simulink library "SMC"  (R2021b)
settings: Solver=VariableStepAuto  StartTime=0.0  StopTime=10.0  RelTol=1e-3
values from neighbouring files (symbols this model uses):
  Ao = At    [SMCDesign_init.m]    (also in SMCDesign_initIA.m)
  Bo = Bv    [SMCDesign_init.m]    (also in SMCDesign_initIA.m)
  CA = pinv(B2)    [SMCCanForm.m]
  Co = Ct    [SMCDesign_init.m]    (also in SMCDesign_initIA.m)
  F = -eye(2)    [Example_init.m]
  Lam_inv = inv(Lam)    [SMCDesign_init.m]    (also in SMCDesign_initIA.m)
  P = lyap(Phi',eye(mm))    [contliaCA2.m]
  To_inv = inv(Tr)    [SMCDesign_init.m]    (also in SMCDesign_initIA.m)
undefined symbols (not defined in the file or in its folder): G, Gl, Gn, P2
libraries: $bdroot x2
settings Model: Creator=lev201  LastModifiedBy=w.schwamm
settings SolverCC: AlgebraicLoopSolver=TrustRegion
settings DataIOCC: ReturnWorkspaceOutputs=off
settings DebuggingCC: SFMachineParentedDataDiag=warning  ArithmeticOperatorsInVariantConditions=warning
settings SFSimCC: SimUseLocalCustomCode=off  CustomCodeUndefinedFunction=UseInterfaceOnly
settings RTWCC: RTWUseLocalCustomCode=off

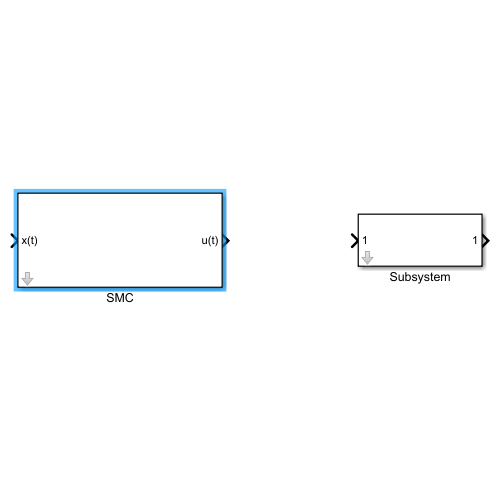
[thumbnail: Simulink's stored preview of the top-level diagram]
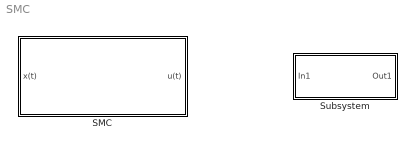
== system SMC ==
  SMC : Subsystem  mask(Sliding Mode Controller){ia=off, obs=off, adpt=off, shs=off, shxo=off, shadpt=off, A=eye(2), B=eye(2), Cc=eye(2), x0=zeros(1,2), obstype=Walcott_Zak, z0=zeros(1,2), Q=eye(2), rho=1, delta=0.01, eps=0, C0=1, PC=1, K0=1, PK=1, Qi=eye(2), Fil=on, Filter=eye(2), FRt=on, rhoo=1, deltao=0.01, epso=0}
      mask prompts: ia "Integral Action"; obs "Observer"; adpt "Adaptive"; shs "Show s(t)"; shxo "Show xo(t)"; shadpt "Show ap(t)"; A "System Matrix (A):"; B "Input Matrix (B):"; Cc "Output Matrix (C):"; x0 "Initial State Vector (x0):"; obstype "Observer Type:"; z0 "Initial State Vector (z0):"; Q "State Weighting Matrix (Q):"; rho "Sliding mode gain (rho):"; delta "Sigmoidal Approximation (delta):"; eps "Boundary Layer Thickness (eps):"; C0 "Initial guess of C:"; PC "Learning rate of C estimator:"; K0 "Initial guess of K:"; PK "Learning rate of K estimator:"; Qi "Integral Action Weighting Matrix (Qi):"; Fil "Pre-Filter Reference Signal"; FRt "Show Filtered R(t)"; rhoo "Sliding mode gain (rhoo):"; deltao "Sigmoidal Approximation (deltao):"; epso "Boundary Layer Thickness (epso):"
      mask help:
      | Sliding Mode Controller with optional observer design
      | Quadratic Minimisation based Sliding Mode Controller with Integral Action
      | If system is over-actuated Control Allocation is automatically used
      mask init:
      | % disp(['shs:' get_param(gcb,'shs')])
      | % clc
      | int=get_param(gcb, 'ia');
      | Shs=get_param(gcb, 'shs');
      | Shxo=get_param(gcb, 'shxo');
      | Fil=get_param(gcb, 'fil');
      | FRT=get_param(gcb, 'FRt');
      | SAD=get_param(gcb, 'shadpt');
      | AD=get_param(gcb, 'adpt');
      | Obs=get_param(gcb, 'obs');
      | 
      | if ~bdIsLibrary(bdroot)
      |     disp('outside lib')
      | else
      |     disp('inside lib')
      | end
      | 
      | [nn mm]=size(B);
      | 
      | % observer is used, if the output matrix does not have full rank
      | % or the flag is set explicitly
      | 
      | % get current number of outports
      | f = Simulink.FindOptions('SearchDepth',1);
      | % num_in=length(Simulink.findBlocksOfType(gcb, 'Inport',f));
      | % num_out=length(Simulink.findBlocksOfType(gcb, 'Outport',f));
      | %fprintf('%d',length(Simulink.findBlocksOfType(gcb, 'Inport',f)))
      | 
      | if strcmp(AD, 'on')
      |     rho=0;
      |     ADPT=1;
      | else
      |     ADPT=0;
      | end
      | 
      | if strcmp(AD, 'on') && strcmp(SAD, 'on')
      |     if strcmp(get_param([gcb '/ap(t)'], 'BlockType'), 'Terminator')
      |         replace([gcb '/ap(t)'], 'built-in/Outport');
      |         num_out=length(Simulink.findBlocksOfType(gcb, 'Outport',f));
      |         set_param([gcb '/ap(t)'],'Port',num2str(num_out));
      |     end
      | else
      |     if strcmp(get_param([gcb '/ap(t)'], 'BlockType'),'Outport')
      |         replace([gcb '/ap(t)'], 'built-in/Terminator')
      |     end
      | end
      | 
      | switch int
      |     case 'off'
      |         [L, P, Lam_inv, S, E, CA,...
      |             Ao, Bo, Co, To_inv, G, F, Gl, Gn, P2]=SMCDesign_init(A, B, Cc, Q);
      |         INTs=0;
      |         ll=size(S,1);
      |         %C=zeros(ll, nn);
      |         L=[zeros(ll, ll) L];
      |         S=[zeros(ll, ll) S];
      |         Sr=zeros(ll, ll);
      |         Lr=[zeros(ll, ll)];
      |         Lrdot=[zeros(ll, ll)];
      |     case 'on'
      |         nn=size(Q,1);
      |         ll=size(Qi,1);
      |         QQ=[Qi zeros(ll, nn)
      |             zeros(nn, ll) Q];
      |         [L, Lr, Lrdot, P, Lam_inv, S, Sr, E, CA, Ao, Bo, Co, To_inv, G, F, Gl, Gn, P2]=SMCDesign_initIA(A, B, Cc, QQ);
      |         INTs=1;
      | end
      | 
      | switch Obs
      |     case 'on'
      | %         if strcmp(get_param([gcb '/x(t)'], 'BlockType'),'Inport')
      | %             replace([gcb '/x(t)'], 'built-in/Ground');
      | %         end
      | %         if strcmp(get_param([gcb '/x(t)'], 'BlockType'), 'Inport')
      | %             set_param([gcb '/x(t)'],'Name','y(t)');
      | %         end
      |         set_param([gcb '/Observer Switch'], 'sw', '1')
      |         %[G,F]=wzobs(At,Bv,Ct);
      |         
      |     case 'off'
      |         %ll=size(S,1);
      |         %G=zeros(ll, ll);
      |         %F=zeros(ll, nn);
      | %         if strcmp(get_param([gcb '/x(t)'], 'BlockType'), 'Ground')
      | %             replace([gcb '/x(t)'], 'built-in/Inport');
      | %             num_in=length(Simulink.findBlocksOfType(gcb, 'Inport',f));
      | %             set_param([gcb '/x(t)'],'Port',num2str(num_in));
      | %         end
      | %         if strcmp(get_param([gcb '/y(t)'], 'BlockType'), 'Inport')
      | %             set_param([gcb '/y(t)'],'Name','x(t)');
      | %         end
      |         set_param([gcb '/Observer Switch'], 'sw', '0')
      | end
      | 
      | % E
      | 
      | switch Shs
      |     case 'on'
      |         if strcmp(get_param([gcb '/s(t)'], 'BlockType'), 'Terminator')
      |             replace([gcb '/s(t)'], 'built-in/Outport');
      |             num_out=length(Simulink.findBlocksOfType(gcb, 'Outport',f));
      |             set_param([gcb '/s(t)'],'Port',num2str(num_out));
      |         end
      |         
      |     case 'off'
      |         if strcmp(get_param([gcb '/s(t)'], 'BlockType'),'Outport')
      |             replace([gcb '/s(t)'], 'built-in/Terminator');
      |         end
      | end
      | 
      | 
      | switch Shxo
      |     case 'on'
      |         if strcmp(get_param([gcb '/xo(t)'], 'BlockType'), 'Terminator')
      |             replace([gcb '/xo(t)'], 'built-in/Outport');
      |             num_out=length(Simulink.findBlocksOfType(gcb, 'Outport',f));
      |             set_param([gcb '/xo(t)'],'Port',num2str(num_out));
      |         end
      |         
      |     case 'off'
      |         if strcmp(get_param([gcb '/xo(t)'], 'BlockType'),'Outport')
      |             replace([gcb '/xo(t)'], 'built-in/Terminator');
      |         end
      | end
      | 
      | switch int
      |     case 'on'
      |         switch Fil
      |             case 'on'
      |                 if strcmp(get_param([gcb '/r(t)'], 'BlockType'),'Inport')
      |                     replace([gcb '/r(t)'], 'built-in/Ground');
      |                 end
      |                 if strcmp(get_param([gcb '/R(t)'], 'BlockType'), 'Ground')
      |                     replace([gcb '/R(t)'], 'built-in/Inport');
      |                     num_in=length(Simulink.findBlocksOfType(gcb, 'Inport',f));
      |                     set_param([gcb '/R(t)'],'Port',num2str(num_in));
      |                 end
      |                 
      |             case 'off'
      |                 if strcmp(get_param([gcb '/R(t)'], 'BlockType'),'Inport')
      |                     replace([gcb '/R(t)'], 'built-in/Ground');
      |                 end
      |                 if strcmp(get_param([gcb '/r(t)'], 'BlockType'), 'Ground')
      |                     replace([gcb '/r(t)'], 'built-in/Inport');
      |                     num_in=length(Simulink.findBlocksOfType(gcb, 'Inport',f));
      |                     set_param([gcb '/r(t)'],'Port',num2str(num_in));
      |                 end
      |         end
      |     case 'off'
      |         replace([gcb '/r(t)'], 'built-in/Ground');
      |         replace([gcb '/R(t)'], 'built-in/Ground');
      | end
      | 
      | if strcmp(Fil, 'on') && strcmp(FRT, 'on') && strcmp(int, 'on')
      |     if strcmp(get_param([gcb '/FR(t)'], 'BlockType'), 'Terminator')
      |         replace([gcb '/FR(t)'], 'built-in/Outport');
      |         num_out=length(Simulink.findBlocksOfType(gcb, 'Outport',f));
      |         set_param([gcb '/FR(t)'],'Port',num2str(num_out));
      |     end
      | else
      |     replace([gcb '/FR(t)'], 'built-in/Terminator')
      | end
      | 
      | if strcmp(Fil, 'on') && strcmp(int, 'on')
      | else
      |     Filter=zeros(ll,ll);
      | end
      mask Callback ia:
      | int = get_param(gcb,'ia');
      | Enables=get_param(gcb, 'MaskEnables');
      | Names=get_param(gcb, 'MaskNames');
      | Vis=get_param(gcb, 'MaskVisibilities');
      | 
      | if strcmp(int,'on')
      |    %Enables{find(strcmp(Names,'Cc'))}='on';
      |    Enables{find(strcmp(Names,'Qi'))}='on';
      |    Enables{find(strcmp(Names,'Fil'))}='on';
      |    Enables{find(strcmp(Names,'Filter'))}='on';
      |    Enables{find(strcmp(Names,'FRt'))}='on';
      | else
      |    %Enables{find(strcmp(Names,'Cc'))}='off';
      |    Enables{find(strcmp(Names,'Qi'))}='off';
      |    Enables{find(strcmp(Names,'Fil'))}='off';
      |    Enables{find(strcmp(Names,'Filter'))}='off';
      |    Enables{find(strcmp(Names,'FRt'))}='off';
      | end
      | set_param(gcb, 'MaskEnables', Enables)
      | set_param(gcb, 'MaskVisibilities', Vis)
      mask Callback obs:
      | val = get_param(gcb,'obs');
      | Enables=get_param(gcb, 'MaskEnables');
      | Names=get_param(gcb, 'MaskNames');
      | Vis=get_param(gcb, 'MaskVisibilities');
      | 
      | if strcmp(val,'on')
      |    Vis{find(strcmp(Names,'shxo'))}='on';
      | else
      |    Vis{find(strcmp(Names,'shxo'))}='off';
      | end
      | set_param(gcb, 'MaskEnables', Enables)
      | set_param(gcb, 'MaskVisibilities', Vis)
      mask Callback adpt:
      | int = get_param(gcb,'adpt');
      | Enables=get_param(gcb, 'MaskEnables');
      | Names=get_param(gcb, 'MaskNames');
      | Vis=get_param(gcb, 'MaskVisibilities');
      | 
      | if strcmp(int,'on')
      |    Vis{find(strcmp(Names,'shadpt'))}='on';
      |    Enables{find(strcmp(Names,'C0'))}='on';
      |    Enables{find(strcmp(Names,'PC'))}='on';
      |    Enables{find(strcmp(Names,'K0'))}='on';
      |    Enables{find(strcmp(Names,'PK'))}='on';
      |    Enables{find(strcmp(Names,'rho'))}='off';
      | else
      |    Vis{find(strcmp(Names,'shadpt'))}='off';
      |    Enables{find(strcmp(Names,'C0'))}='off';
      |    Enables{find(strcmp(Names,'PC'))}='off';
      |    Enables{find(strcmp(Names,'K0'))}='off';
      |    Enables{find(strcmp(Names,'PK'))}='off';
      |    Enables{find(strcmp(Names,'rho'))}='on';
      | end
      | set_param(gcb, 'MaskEnables', Enables)
      | set_param(gcb, 'MaskVisibilities', Vis)
      mask TypeOptions obstype: Walcott_Zak | Discontinuous
      mask Callback obstype:
      | % Get the mask parameter values. This is a cell
      | %   array of character vectors.
      | maskStr = get_param(gcb,'obstype');
      | 
      | % The pop-up menu is the first mask parameter.
      | %   Check the value selected in the pop-up
      | if strcmp(maskStr(1),'W'),
      |     % Walcott-Zak Observer (G, F)
      |     set_param([gcb '/WZ_DIS'], 'sw', '1');
      | 
      | else
      |     % Discontinuous Observer (Gl, Gn, P2)
      |     set_param([gcb '/WZ_DIS'], 'sw', '0')
      | end
      mask Callback Fil:
      | FIL = get_param(gcb,'Fil');
      | Enables=get_param(gcb, 'MaskEnables');
      | Names=get_param(gcb, 'MaskNames');
      | Vis=get_param(gcb, 'MaskVisibilities');
      | 
      | if strcmp(FIL,'on')
      |    Vis{find(strcmp(Names,'Filter'))}='on';
      |    Vis{find(strcmp(Names,'FRt'))}='on';
      | else
      |    Vis{find(strcmp(Names,'Filter'))}='off';
      |    Vis{find(strcmp(Names,'FRt'))}='off';
      | end
      | 
      | set_param(gcb, 'MaskEnables', Enables)
      | set_param(gcb, 'MaskVisibilities', Vis)
      mask DialogControl Container4 Prompt: Controller Configuration
      mask DialogControl shxo Tooltip: Show Observer States
      mask DialogControl shadpt Tooltip: Show Adaptive Parameters
      mask DialogControl Container3 Prompt: Model Parameters
      mask DialogControl Container17 Prompt: Observer Parameters
      mask DialogControl Container7 Prompt: Controller
      mask DialogControl Container16 Prompt: Fixed Parameters
      mask DialogControl Container12 Prompt: Adaptive Parameters
      mask DialogControl Container9 Prompt: Integral Action
      mask DialogControl Container14 Prompt: Observer
      mask DialogControl Container18 Prompt: Fixed Parameters
  Subsystem : Subsystem
      mask init:
      | if ~bdIsLibrary(bdroot)
      |     disp('outside lib')
      | else
      |     disp('inside lib')
      | end
      mask DialogControl button Prompt: Initialize
      mask DialogControl button Callback: set_param(gcs,'SimulationCommand','Update')

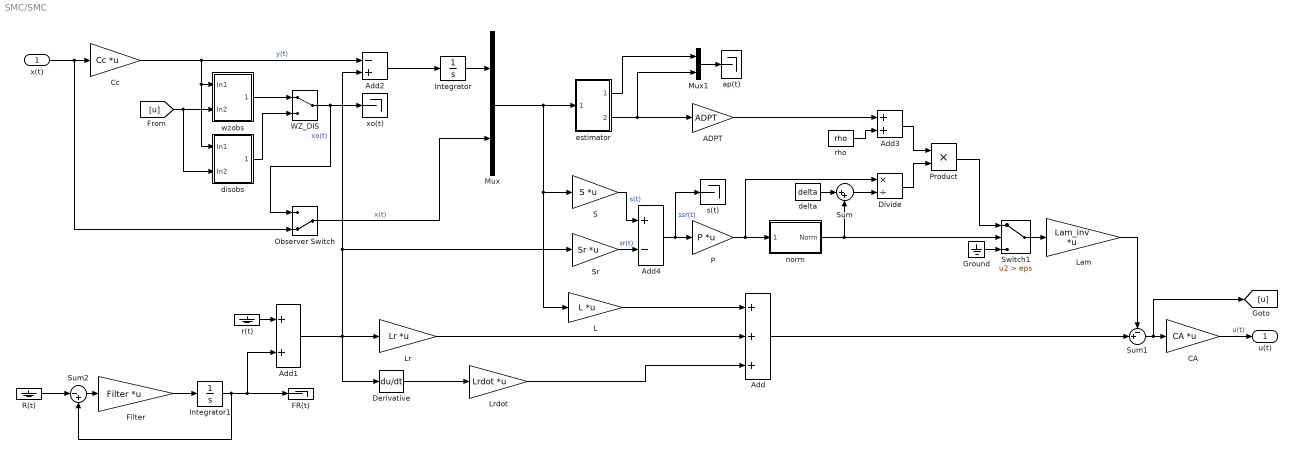
== system SMC/SMC ==
  x(t) : Inport
  ADPT : Gain  Gain=ADPT
  Add : Sum  Inputs=+++
  Add1 : Sum
  Add2 : Sum  Inputs=-+
  Add3 : Sum
  Add4 : Sum  Inputs=+-
  CA : Gain  Gain=CA  Multiplication=Matrix(K*u) (u vector)
  Cc : Gain  Gain=Cc  Multiplication=Matrix(K*u) (u vector)
  Derivative : Derivative
  Divide : Product  Inputs=*/
  FR(t) : Terminator
  Filter : Gain  Gain=Filter  Multiplication=Matrix(K*u) (u vector)
  Ground : Ground
  Integrator : Integrator
  Integrator1 : Integrator
  L : Gain  Gain=L  Multiplication=Matrix(K*u) (u vector)
  Lam : Gain  Gain=Lam_inv  Multiplication=Matrix(K*u) (u vector)
  Lr : Gain  Gain=Lr  Multiplication=Matrix(K*u) (u vector)
  Lrdot : Gain  Gain=Lrdot  Multiplication=Matrix(K*u) (u vector)
  Mux : Mux  Inputs=2
  Mux1 : Mux  Inputs=2
  Observer Switch : ManualSwitch  CurrentSetting=0
  P : Gain  Gain=P  Multiplication=Matrix(K*u) (u vector)
  Product : Product
  R(t) : Ground
  S : Gain  Gain=S  Multiplication=Matrix(K*u) (u vector)
  Sr : Gain  Gain=Sr  Multiplication=Matrix(K*u) (u vector)
  Sum : Sum  Inputs=|++
  Sum1 : Sum  Inputs=-+|
  Sum2 : Sum  Inputs=|-+
  Switch1 : Switch  Criteria=u2 > Threshold  Threshold=eps  ZeroCross=off
  WZ_DIS : ManualSwitch
  ap(t) : Terminator
  delta : Constant  Value=delta
  disobs : Subsystem
  estimator : Subsystem
  norm : Subsystem
  r(t) : Ground
  rho : Constant  Value=rho
  s(t) : Terminator
  wzobs : Subsystem
  xo(t) : Terminator
  u(t) : Outport  VectorParamsAs1DForOutWhenUnconnected=off
  wires:
  Add/1 -> Sum1/2
  norm/1(Norm) -> Sum/2, Switch1/2
  P/1 -> Divide/1, norm/1(Vector)
  Divide/1 -> Product/2
  CA/1 -> u(t)/1  "u(t)"
  Sum1/1 -> [u], CA/1
  Add4/1 -> s(t)/1, P/1  "ssr(t)"
  Add2/1 -> Integrator/1
  Integrator/1 -> Mux/1
  L/1 -> Add/1
  Sum/1 -> Divide/2
  delta/1 -> Sum/1
  Lr/1 -> Add/2
  Mux/1 -> L/1, S/1, estimator/1(x(t))
  r(t)/1 -> Add1/1
  Add1/1 -> Sr/1, Add2/2, Lr/1, Derivative/1
  R(t)/1 -> Sum2/1
  Sum2/1 -> Filter/1
  Integrator1/1 -> Sum2/2, FR(t)/1, Add1/2
  Filter/1 -> Integrator1/1
  Ground/1 -> Switch1/3
  Switch1/1 -> Lam/1
  estimator/1(est-par) -> Mux1/1
  Mux1/1 -> ap(t)/1
  estimator/2(rho) -> ADPT/1, Mux1/2
  Add3/1 -> Product/1
  rho/1 -> Add3/2
  ADPT/1 -> Add3/1
  Product/1 -> Switch1/1
  Lam/1 -> Sum1/1
  Sr/1 -> Add4/2  "sr(t)"
  S/1 -> Add4/1  "s(t)"
  Derivative/1 -> Lrdot/1
  Lrdot/1 -> Add/3
  Observer Switch/1 -> Mux/2  "x(t)"
  [u] -> disobs/2(In2), wzobs/2(In2)
  disobs/1(Out1) -> WZ_DIS/2
  wzobs/1(Out1) -> WZ_DIS/1
  WZ_DIS/1 -> Observer Switch/1, xo(t)/1  "xo(t)"
  x(t)/1 -> Observer Switch/2, Cc/1
  Cc/1 -> Add2/1, wzobs/1(In1), disobs/1(In1)  "y(t)"

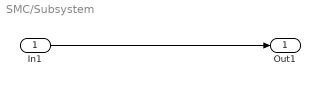
== system SMC/Subsystem ==
  In1 : Inport
  Out1 : Outport
  wires:
  In1/1 -> Out1/1

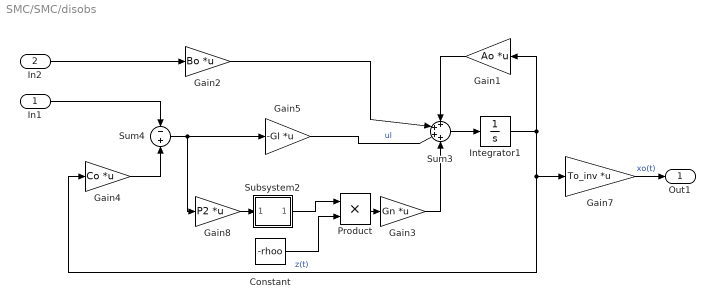
== system SMC/SMC/disobs ==
  In1 : Inport
  In2 : Inport  Port=2
  Constant : Constant  Value=-rhoo  SampleTime=-1
  Gain1 : Gain  Gain=Ao  Multiplication=Matrix(K*u)
  Gain2 : Gain  Gain=Bo  Multiplication=Matrix(K*u)
  Gain3 : Gain  Gain=Gn  Multiplication=Matrix(K*u)
  Gain4 : Gain  Gain=Co  Multiplication=Matrix(K*u)
  Gain5 : Gain  Gain=-Gl  Multiplication=Matrix(K*u)
  Gain7 : Gain  Gain=To_inv  Multiplication=Matrix(K*u)
  Gain8 : Gain  Gain=P2  Multiplication=Matrix(K*u)
  Integrator1 : Integrator  InitialCondition=z0
  Product : Product
  Subsystem2 : Subsystem  mask{delta=deltao}
      mask prompts: delta "Unit vector delta:"
      mask Display: disp('UnV')
  Sum3 : Sum  Inputs=++++
  Sum4 : Sum  Inputs=-+
  Out1 : Outport
  wires:
  In1/1 -> Sum4/1
  In2/1 -> Gain2/1
  Sum3/1 -> Integrator1/1
  Gain1/1 -> Sum3/1
  Gain3/1 -> Sum3/4
  Gain8/1 -> Subsystem2/1(In1)
  Gain2/1 -> Sum3/2
  Gain4/1 -> Sum4/2
  Integrator1/1 -> Gain4/1, Gain7/1, Gain1/1  "z(t)"
  Sum4/1 -> Gain8/1, Gain5/1
  Gain5/1 -> Sum3/3  "ul"
  Gain7/1 -> Out1/1  "xo(t)"
  Constant/1 -> Product/2
  Product/1 -> Gain3/1
  Subsystem2/1(Out1) -> Product/1

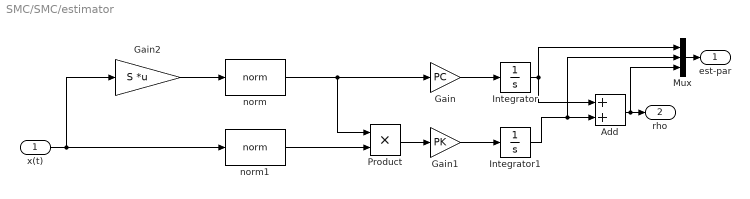
== system SMC/SMC/estimator ==
  x(t) : Inport
  Add : Sum
  Gain : Gain  Gain=PC
  Gain1 : Gain  Gain=PK
  Gain2 : Gain  Gain=S  Multiplication=Matrix(K*u) (u vector)
  Integrator : Integrator  InitialCondition=C0
  Integrator1 : Integrator  InitialCondition=K0
  Mux : Mux  Inputs=3
  Product : Product
  norm : $bdroot/SMC/norm  SystemSampleTime=-1  VariantActivationTime=update diagram  Latency=0  AutoFrameSizeCalculation=off
  norm1 : $bdroot/SMC/norm  SystemSampleTime=-1  VariantActivationTime=update diagram  Latency=0  AutoFrameSizeCalculation=off
  est-par : Outport  VectorParamsAs1DForOutWhenUnconnected=off
  rho : Outport  Port=2  VectorParamsAs1DForOutWhenUnconnected=off
  wires:
  Gain/1 -> Integrator/1
  Integrator/1 -> Add/1, Mux/1
  norm/1 -> Product/1, Gain/1
  x(t)/1 -> norm1/1, Gain2/1
  norm1/1 -> Product/2
  Product/1 -> Gain1/1
  Gain1/1 -> Integrator1/1
  Add/1 -> Mux/3, rho/1
  Integrator1/1 -> Mux/2, Add/2
  Gain2/1 -> norm/1
  Mux/1 -> est-par/1

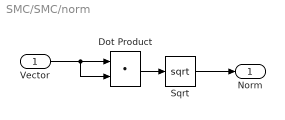
== system SMC/SMC/norm ==
  Vector : Inport
  Dot Product : DotProduct  InputSameDT=on  OutDataTypeStr=Inherit: Inherit via internal rule
  Sqrt : Sqrt  SaturateOnIntegerOverflow=on
  Norm : Outport  VectorParamsAs1DForOutWhenUnconnected=off
  wires:
  Dot Product/1 -> Sqrt/1
  Vector/1 -> Dot Product/2, Dot Product/1
  Sqrt/1 -> Norm/1

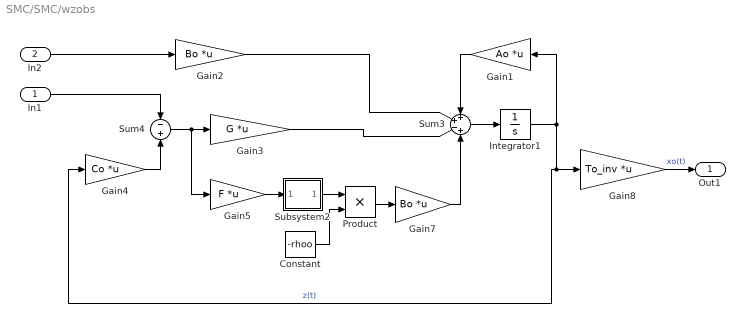
== system SMC/SMC/wzobs ==
  In1 : Inport
  In2 : Inport  Port=2
  Constant : Constant  Value=-rhoo  SampleTime=-1
  Gain1 : Gain  Gain=Ao  Multiplication=Matrix(K*u) (u vector)
  Gain2 : Gain  Gain=Bo  Multiplication=Matrix(K*u) (u vector)
  Gain3 : Gain  Gain=G  Multiplication=Matrix(K*u) (u vector)
  Gain4 : Gain  Gain=Co  Multiplication=Matrix(K*u) (u vector)
  Gain5 : Gain  Gain=F  Multiplication=Matrix(K*u) (u vector)
  Gain7 : Gain  Gain=Bo  Multiplication=Matrix(K*u) (u vector)
  Gain8 : Gain  Gain=To_inv  Multiplication=Matrix(K*u) (u vector)
  Integrator1 : Integrator  InitialCondition=z0
  Product : Product
  Subsystem2 : Subsystem  mask{delta=deltao}
      mask prompts: delta "Unit vector delta:"
      mask Display: disp('UnV')
  Sum3 : Sum  Inputs=++-+
  Sum4 : Sum  Inputs=-+
  Out1 : Outport
  wires:
  Sum4/1 -> Gain5/1, Gain3/1
  Integrator1/1 -> Gain4/1, Gain8/1, Gain1/1  "z(t)"
  Gain4/1 -> Sum4/2
  Gain2/1 -> Sum3/2
  Product/1 -> Gain7/1
  Gain5/1 -> Subsystem2/1(In1)
  Subsystem2/1(Out1) -> Product/1
  Gain7/1 -> Sum3/4
  Gain3/1 -> Sum3/3
  Gain1/1 -> Sum3/1
  Sum3/1 -> Integrator1/1
  In2/1 -> Gain2/1
  In1/1 -> Sum4/1
  Constant/1 -> Product/2
  Gain8/1 -> Out1/1  "xo(t)"

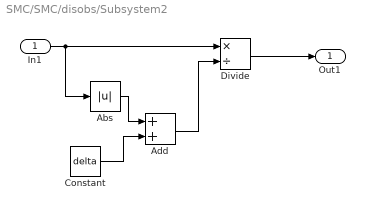
== system SMC/SMC/disobs/Subsystem2 ==
  In1 : Inport
  Abs : Abs  ZeroCross=off
  Add : Sum
  Constant : Constant  Value=delta  SampleTime=-1
  Divide : Product  Inputs=*/
  Out1 : Outport
  wires:
  In1/1 -> Abs/1, Divide/1
  Divide/1 -> Out1/1
  Abs/1 -> Add/1
  Add/1 -> Divide/2
  Constant/1 -> Add/2

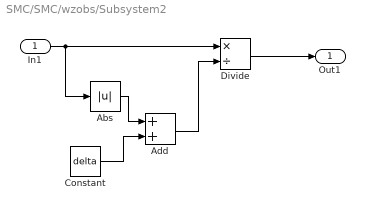
== system SMC/SMC/wzobs/Subsystem2 ==
  In1 : Inport
  Abs : Abs  ZeroCross=off
  Add : Sum
  Constant : Constant  Value=delta  SampleTime=-1
  Divide : Product  Inputs=*/
  Out1 : Outport
  wires:
  Constant/1 -> Add/2
  Add/1 -> Divide/2
  Abs/1 -> Add/1
  Divide/1 -> Out1/1
  In1/1 -> Divide/1, Abs/1
